simulink model "SimulationOne"  (R2023b)
settings: Solver=VariableStepAuto  StartTime=0.0  StopTime=10.0  RelTol=1e-3
libraries: simulink x2
settings Model: Creator=jsonm  LastModifiedBy=jsonm

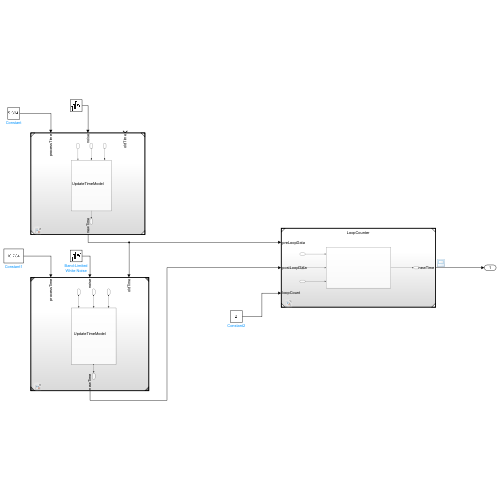
[thumbnail: Simulink's stored preview of the top-level diagram]
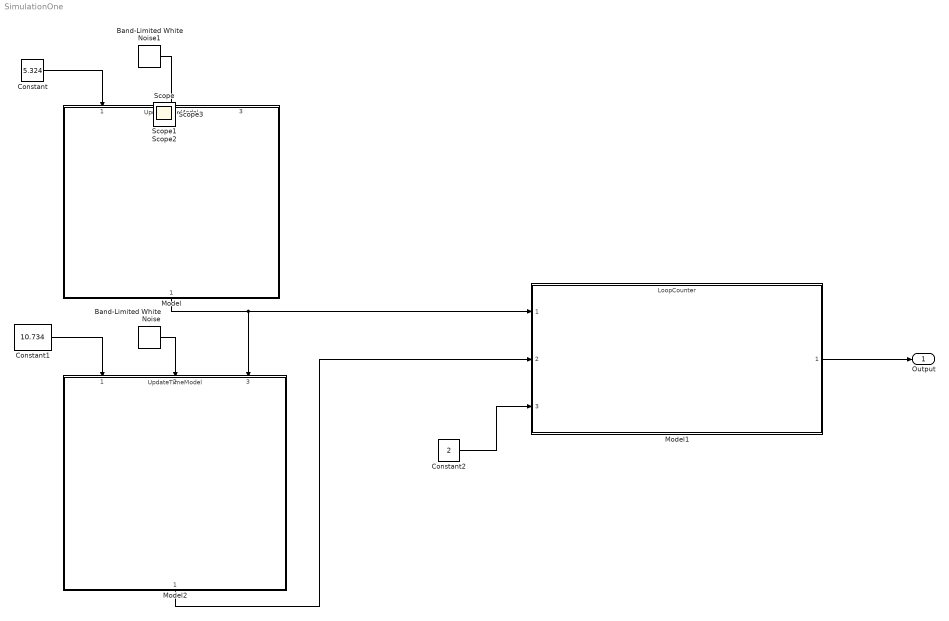
== system SimulationOne ==
  Band-Limited White Noise : simulink/Sources/Band-Limited White Noise  Cov=[0.1]  Ts=0.1  seed=[23341]
  Band-Limited White Noise1 : simulink/Sources/Band-Limited White Noise  Cov=[0.1]  Ts=0.1  seed=[23341]
  Constant : Constant  Value=5.324
  Constant1 : Constant  Value=10.734
  Constant2 : Constant  Value=2
  Model : ModelReference  ModelNameDialog=UpdateTimeModel.slx  SimulationMode=Normal  ModelReferenceVersion=1.1
  Model1 : ModelReference  ModelNameDialog=LoopCounter.slx  SimulationMode=Normal  ModelReferenceVersion=1.1
  Model2 : ModelReference  ModelNameDialog=UpdateTimeModel.slx  SimulationMode=Normal  ModelReferenceVersion=1.1
  Output : Outport
  Scope{,1..3} (4 alike) : Scope
  wires:
  Model/1 -> Model2/3, Model1/1
  Model2/1 -> Model1/2
  Constant2/1 -> Model1/3
  Model1/1 -> Output/1
  Band-Limited White Noise1/1 -> Model/2
  Constant/1 -> Model/1
  Band-Limited White Noise/1 -> Model2/2
  Constant1/1 -> Model2/1
